simulink model "regulation"  (R2013a)
settings: Solver=VariableStepDiscrete  StartTime=0.0  StopTime=30  RelTol=1e-3
model workspace (MAT data in the model file):
  Kig = 0.005
  Kp = 0.01
undefined symbols (not defined in the file): DiscIntNeverNeededParam
settings Model: Creator=Penultimo  LastModifiedBy=Penultimo
settings RTWCC: TargetLang=C++

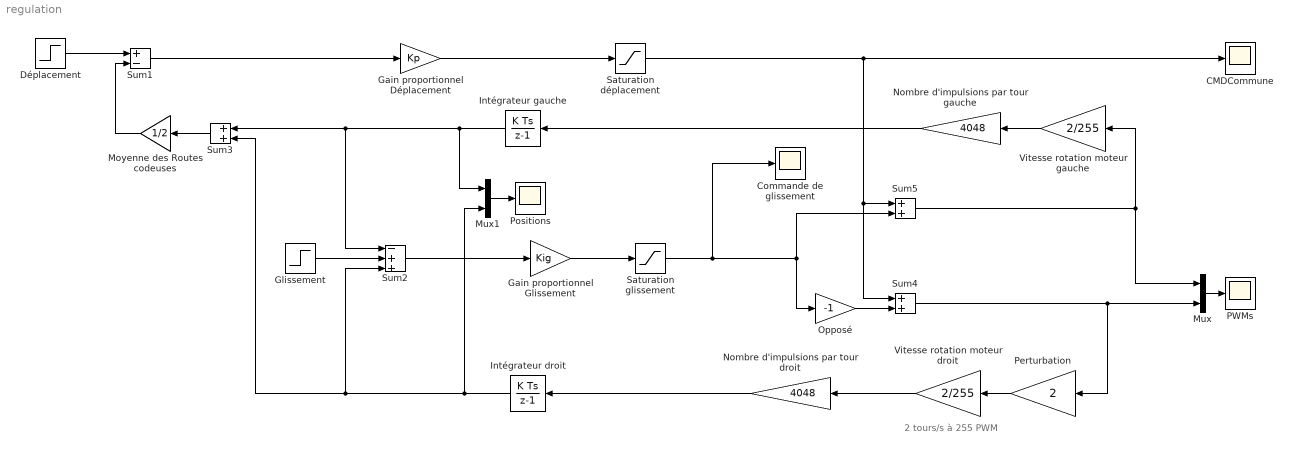
== system regulation ==
  note: 2 tours/s à 255 PWM
  CMDCommune : Scope
      settings: TimeRange=0.003142278523873276  YMin=0.1990895173987563  YMax=0.1999770183952487  SaveName=ScopeData2
  Commande de glissement : Scope
      settings: TimeRange=0.003142278523873276  YMin=0.1990895173987563  YMax=0.1999770183952487
  Déplacement : Step  After=0  SampleTime=0
  Gain proportionnel Déplacement : Gain  Gain=Kp  SampleTime=0.01  SaturateOnIntegerOverflow=on  OutDataTypeStr=Inherit: Same as input  ParamDataTypeStr=Inherit: Same as input
  Gain proportionnel Glissement : Gain  Gain=Kig  SampleTime=0.01  SaturateOnIntegerOverflow=on  OutDataTypeStr=Inherit: Same as input  ParamDataTypeStr=Inherit: Same as input
  Glissement : Step  After=25000  SampleTime=0
  Intégrateur droit : DiscreteIntegrator  SampleTime=0.01  ICPrevOutput=DiscIntNeverNeededParam  ICPrevScaledInput=DiscIntNeverNeededParam
  Intégrateur gauche : DiscreteIntegrator  SampleTime=0.01  ICPrevOutput=DiscIntNeverNeededParam  ICPrevScaledInput=DiscIntNeverNeededParam
  Moyenne des Routes codeuses : Gain  Gain=1/2  SampleTime=0.01  SaturateOnIntegerOverflow=on  OutDataTypeStr=Inherit: Same as input  ParamDataTypeStr=Inherit: Same as input
  Mux : Mux  Inputs=2
  Mux1 : Mux  Inputs=2
  Nombre d'impulsions par tour droit : Gain  Gain=4048  SampleTime=0.01  SaturateOnIntegerOverflow=on  OutDataTypeStr=Inherit: Same as input  ParamDataTypeStr=Inherit: Same as input
  Nombre d'impulsions par tour gauche : Gain  Gain=4048  SampleTime=0.01  SaturateOnIntegerOverflow=on  OutDataTypeStr=Inherit: Same as input  ParamDataTypeStr=Inherit: Same as input
  Opposé : Gain  Gain=-1  SampleTime=0.01  SaturateOnIntegerOverflow=on  OutDataTypeStr=Inherit: Same as input  ParamDataTypeStr=Inherit: Same as input
  PWMs : Scope
      settings: TimeRange=50  YMin=0  YMax=140  SaveName=ScopeData4
  Perturbation : Gain  Gain=2  SampleTime=0.01  SaturateOnIntegerOverflow=on  OutDataTypeStr=Inherit: Same as input  ParamDataTypeStr=Inherit: Same as input
  Positions : Scope
      settings: TimeRange=0.003142278523873276  YMin=0.1990895173987563  YMax=0.1999770183952487  SaveName=ScopeData5
  Saturation déplacement : Saturate  UpperLimit=125  LowerLimit=-125  SampleTime=0.01
  Saturation glissement : Saturate  UpperLimit=125  LowerLimit=-125  SampleTime=0.01
  Sum1 : Sum  Inputs=+-  SampleTime=0.01  SaturateOnIntegerOverflow=on  InputSameDT=on  OutDataTypeStr=Inherit: Same as first input
  Sum2 : Sum  Inputs=-++  SampleTime=0.01  SaturateOnIntegerOverflow=on  InputSameDT=on  OutDataTypeStr=Inherit: Same as first input
  Sum3 : Sum  SampleTime=0.01  SaturateOnIntegerOverflow=on  InputSameDT=on  OutDataTypeStr=Inherit: Same as first input
  Sum4 : Sum  SampleTime=0.01  SaturateOnIntegerOverflow=on  InputSameDT=on  OutDataTypeStr=Inherit: Same as first input
  Sum5 : Sum  SampleTime=0.01  SaturateOnIntegerOverflow=on  InputSameDT=on  OutDataTypeStr=Inherit: Same as first input
  Vitesse rotation moteur droit : Gain  Gain=2/255  SampleTime=0.01  SaturateOnIntegerOverflow=on  OutDataTypeStr=Inherit: Same as input  ParamDataTypeStr=Inherit: Same as input
  Vitesse rotation moteur gauche : Gain  Gain=2/255  SampleTime=0.01  SaturateOnIntegerOverflow=on  OutDataTypeStr=Inherit: Same as input  ParamDataTypeStr=Inherit: Same as input
  wires:
  Déplacement/1 -> Sum1/1
  Moyenne des Routes codeuses/1 -> Sum1/2
  Sum3/1 -> Moyenne des Routes codeuses/1
  Sum2/1 -> Gain proportionnel Glissement/1
  Sum1/1 -> Gain proportionnel Déplacement/1
  Gain proportionnel Glissement/1 -> Saturation glissement/1
  Nombre d'impulsions par tour gauche/1 -> Intégrateur gauche/1
  Gain proportionnel Déplacement/1 -> Saturation déplacement/1
  Sum4/1 -> Perturbation/1, Mux/2
  Saturation déplacement/1 -> Sum4/1, Sum5/1, CMDCommune/1
  Vitesse rotation moteur gauche/1 -> Nombre d'impulsions par tour gauche/1
  Vitesse rotation moteur droit/1 -> Nombre d'impulsions par tour droit/1
  Sum5/1 -> Vitesse rotation moteur gauche/1, Mux/1
  Intégrateur gauche/1 -> Mux1/1, Sum2/1, Sum3/1
  Intégrateur droit/1 -> Mux1/2, Sum2/3, Sum3/2
  Saturation glissement/1 -> Commande de glissement/1, Sum5/2, Opposé/1
  Opposé/1 -> Sum4/2
  Nombre d'impulsions par tour droit/1 -> Intégrateur droit/1
  Perturbation/1 -> Vitesse rotation moteur droit/1
  Glissement/1 -> Sum2/2
  Mux/1 -> PWMs/1
  Mux1/1 -> Positions/1
